simulink model "Prac02_2_1"  (R2015a)
settings: Solver=ode45  StartTime=0.0  StopTime=8  RelTol=1e-3
settings Model: Creator=redes  LastModifiedBy=redes

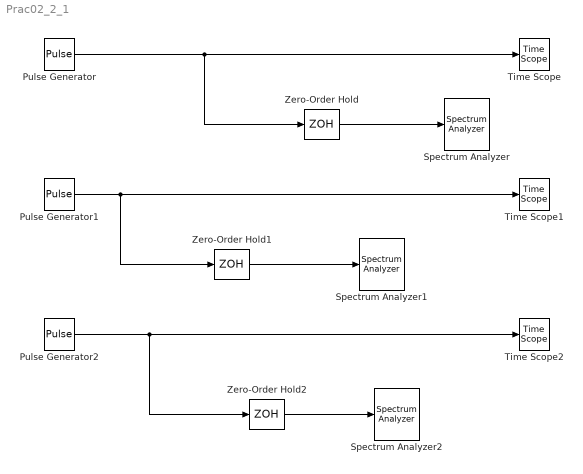
== system Prac02_2_1 ==
  Pulse Generator : DiscretePulseGenerator  PulseType=Time based  Period=1  PulseWidth=50
  Pulse Generator1 : DiscretePulseGenerator  PulseType=Time based  Period=0.5  PulseWidth=50
  Pulse Generator2 : DiscretePulseGenerator  PulseType=Time based  Period=0.25  PulseWidth=50
  Spectrum Analyzer : SpectrumAnalyzer
  Spectrum Analyzer1 : SpectrumAnalyzer
  Spectrum Analyzer2 : SpectrumAnalyzer
  Time Scope : TimeScope  DefaultConfigurationName=spbscopes.TimeScopeBlockCfg
  Time Scope1 : TimeScope  DefaultConfigurationName=spbscopes.TimeScopeBlockCfg
  Time Scope2 : TimeScope  DefaultConfigurationName=spbscopes.TimeScopeBlockCfg
  Zero-Order Hold : ZeroOrderHold  SampleTime=0.0025
  Zero-Order Hold1 : ZeroOrderHold  SampleTime=0.0025
  Zero-Order Hold2 : ZeroOrderHold  SampleTime=0.0025
  wires:
  Zero-Order Hold/1 -> Spectrum Analyzer/1
  Pulse Generator/1 -> Zero-Order Hold/1, Time Scope/1
  Zero-Order Hold1/1 -> Spectrum Analyzer1/1
  Pulse Generator1/1 -> Zero-Order Hold1/1, Time Scope1/1
  Zero-Order Hold2/1 -> Spectrum Analyzer2/1
  Pulse Generator2/1 -> Zero-Order Hold2/1, Time Scope2/1
